simulink model "known_parameters"  (R2021a)
settings: Solver=VariableStepAuto  StartTime=0.0  StopTime=20.0  RelTol=1e-3
libraries: simulink x1
settings Model: Creator=tejal  LastModifiedBy=dhruv

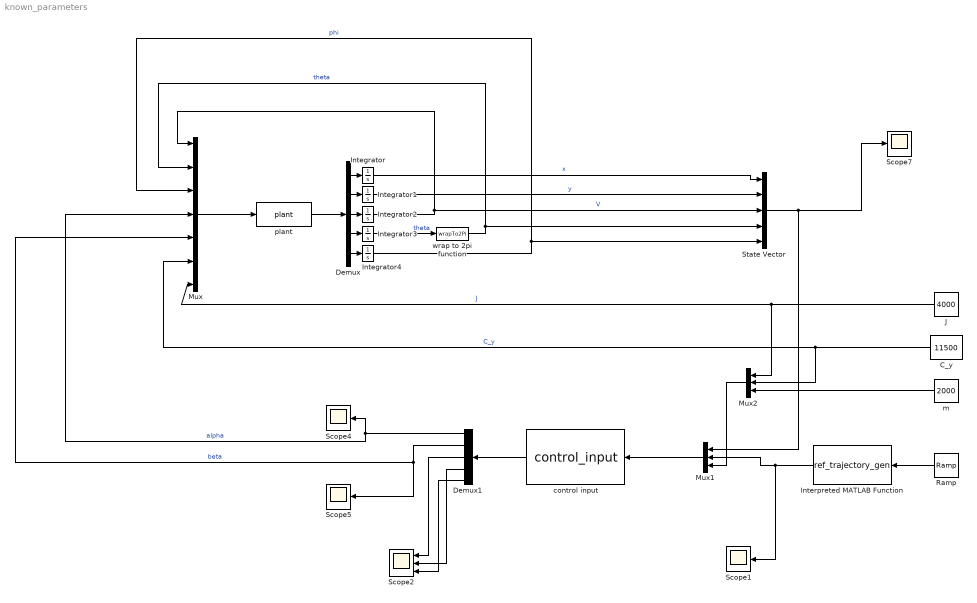
== system known_parameters ==
  C_y : Constant  Value=11500
  Demux : Demux  Outputs=5
  Demux1 : Demux  Outputs=5
  Integrator : Integrator  InitialCondition=0.00005
  Integrator1 : Integrator  InitialCondition=0.00000005
  Integrator2 : Integrator  InitialCondition=1
  Integrator3 : Integrator
  Integrator4 : Integrator
  Interpreted MATLAB Function : MATLABFcn  MATLABFcn=ref_trajectory_gen  OutputDimensions=7
  J : Constant  Value=4000
  Mux : Mux  Inputs=7
  Mux1 : Mux  Inputs=3
  Mux2 : Mux  Inputs=3
  Ramp : simulink/Sources/Ramp  slope=1  start=0  InitialOutput=0
  Scope{1,4..5,7} (4 alike) : Scope
  Scope2 : Scope  NumInputPorts=3
  State Vector : Mux  Inputs=5
  control input : MATLABFcn  MATLABFcn=control_input  OutputDimensions=5
  m : Constant  Value=2000
  plant : MATLABFcn  MATLABFcn=plant  OutputDimensions=5
  wrap to 2pi function : MATLABFcn  MATLABFcn=wrapTo2Pi
  wires:
  Mux/1 -> plant/1
  plant/1 -> Demux/1
  Demux/1 -> Integrator/1
  Demux/5 -> Integrator4/1
  Demux/4 -> Integrator3/1
  Demux/3 -> Integrator2/1
  Demux/2 -> Integrator1/1
  Integrator/1 -> State Vector/1  "x"
  Integrator1/1 -> State Vector/2  "y"
  Integrator2/1 -> Mux/1, State Vector/3  "V"
  Integrator3/1 -> wrap to 2pi function/1  "theta"
  Integrator4/1 -> State Vector/5, Mux/3  "phi"
  J/1 -> Mux2/1, Mux/7  "J"
  C_y/1 -> Mux2/2, Mux/6  "C_y"
  State Vector/1 -> Mux1/1, Scope7/1
  Demux1/2 -> Scope5/1, Mux/5  "beta"
  Demux1/1 -> Mux/4, Scope4/1  "alpha"
  wrap to 2pi function/1 -> State Vector/4, Mux/2  "theta"
  control input/1 -> Demux1/1
  Ramp/1 -> Interpreted MATLAB Function/1
  Interpreted MATLAB Function/1 -> Scope1/1, Mux1/2
  Mux1/1 -> control input/1
  m/1 -> Mux2/3
  Mux2/1 -> Mux1/3
  Demux1/3 -> Scope2/1
  Demux1/4 -> Scope2/2
  Demux1/5 -> Scope2/3
